simulink library "snn_champions_lib"  (R2026a)
settings: Solver=VariableStepAuto
(part 4 of 24)

== matlab function snn_champions_lib/Michelangelo/SNN ==
  data: x_phys input; params output
function params = SNN(x_phys)
%#codegen
% Blocco champion SELF-CONTAINED: pesi bakati + forward ALIF + decode, zero dipendenze .m.
  W_IN  = [0.5 -0.5 -0.25 2;-1 0.5 -1 2;0.25 -2 1 0.5;0.5 0.25 0.125 -0.25;0.5 -0.5 -0.125 1;-1 1 -1 1;-1 -0.5 0.5 0.5;0.5 0.5 1 -1;-0.25 -0.125 -1 2;-0.5 2 0.25 -0.0625;-0.5 0.0625 0.25 1;0.25 -1 1 1;1 0.5 -0.25 0.125;-2 2 0.5 -0.25;-0.5 1 0.25 -0.5;-0.5 -0.25 1 -1;1 -0.125 0.5 -0.25;0.125 -0.25 2 -0.0625;2 0.0625 -0.25 1;-2 0.5 -0.125 2;0.5 -0.5 1 -0.5;1 0 2 -0.25;-0.25 1 0.25 0.25;1 2 -0.5 -0.125;2 1 -0.5 -0.125;-1 2 0.25 -0.125;0.5 0.5 -0.25 1;-0.5 -0.5 2 -0.0625;1 -0.5 -0.125 0.5;1 -0.0625 0.125 0.5;-0.25 1 0.25 -0.5;-1 1 0.25 0.125];
  U     = [0.125 0 0.0625 0.0625 -0.0625 -0.125 0 0 0.0625 0.0625 0 0.125 0.125 0.0625 -0.125 -0.0625;0 -0.0625 0.0625 -0.0625 0 -0.125 0.0625 -0.0625 0.0625 -0.0625 0 -0.125 0.0625 -0.0625 -0.0625 0;0.0625 0.125 -0.0625 0.0625 0.0625 0.0625 0.0625 0 -0.0625 0 0 0 0.0625 0 0 0.0625;0 0.0625 -0.0625 0.0625 0 -0.0625 0 0 0.0625 -0.0625 -0.0625 0 0.125 0.0625 -0.0625 0.0625;-0.0625 0.0625 0.0625 0 -0.0625 0 -0.0625 0.0625 -0.0625 -0.0625 0 -0.125 0 0.0625 0 0;-0.0625 0.125 -0.125 0 0.0625 -0.125 0.0625 0 0.0625 -0.125 0 -0.0625 0.125 -0.125 -0.125 0;0 -0.0625 -0.125 0 0.125 0.0625 0.0625 0.125 0 -0.0625 -0.0625 0.125 0 -0.125 0 0;-0.0625 0.125 -0.0625 0.125 0.0625 -0.25 0 -0.0625 -0.125 -0.125 -0.125 0.0625 0.0625 -0.125 -0.125 0;0 0.0625 0.0625 -0.125 -0.125 0 0 0 0 -0.0625 -0.0625 0 0 -0.0625 -0.0625 0;0 -0.0625 -0.0625 -0.125 -0.0625 -0.0625 0.0625 0 -0.0625 -0.0625 0 -0.0625 0 0.0625 0 -0.125;0 0.0625 0 -0.125 0 0 -0.0625 0.0625 0 -0.0625 0.0625 0.0625 -0.0625 -0.0625 -0.0625 0.0625;0 0.125 -0.125 0 0.125 0 -0.0625 0.125 -0.125 -0.0625 0 0.0625 0 0 0.0625 0;0 0 0 0 -0.0625 0.0625 0 0.125 0.125 -0.125 0 0.0625 0.0625 0.0625 -0.125 0;-0.0625 0 -0.0625 0 -0.0625 -0.0625 0 -0.25 0 -0.125 0 0.25 0.125 -0.0625 -0.125 0.25;0.0625 0 -0.0625 0 0 -0.0625 0 0 -0.0625 -0.0625 0 0.125 0.125 -0.0625 -0.0625 -0.25;0 0 0.0625 -0.0625 0.0625 -0.125 0.0625 0 0 0.0625 -0.0625 0 0 -0.125 0.0625 0;-0.0625 0.0625 -0.125 0.125 0 -0.125 0.125 0 -0.0625 -0.0625 -0.125 0.0625 0.25 -0.0625 -0.125 -0.125;0 0.0625 -0.0625 0 0 0 0 -0.0625 0 0 -0.0625 0 0 -0.0625 0 0;0 0 0 -0.0625 0 -0.0625 0 0.125 0 -0.0625 0.0625 0 0.125 0.0625 0 -0.125;0.0625 0 0.0625 -0.0625 -0.0625 0 0.25 0.125 0.125 -0.125 -0.125 -0.0625 -0.0625 -0.0625 -0.0625 0.0625;0.125 -0.0625 -0.0625 -0.0625 0.125 0.0625 0 0.0625 -0.0625 0 -0.0625 0.0625 0 0.25 0.0625 0.125;0.0625 0.125 0.125 0.0625 -0.0625 0 0 0 0.125 0 0.0625 0.0625 0 0 0 0.0625;0.25 0 -0.0625 0 -0.125 0.0625 0.125 0 0.0625 -0.125 0 0.0625 -0.25 0.125 0 0.125;0.0625 -0.0625 -0.125 0 -0.125 -0.125 0 0.125 0 0 0 0.25 0 -0.0625 -0.125 0.25;0 -0.125 -0.125 0.125 -0.125 0 0 0.0625 0.125 -0.125 -0.0625 -0.0625 0.125 -0.0625 0.0625 -0.125;-0.0625 0 0.0625 -0.0625 0 -0.25 0 0.0625 0 -0.0625 0 -0.0625 0.0625 0.0625 0.0625 -0.25;0.0625 0.125 -0.0625 0.0625 -0.0625 0.125 0.0625 0.0625 0.0625 -0.0625 0.125 0.0625 -0.0625 -0.0625 0 0;0.0625 0.0625 0 0.125 -0.125 0 -0.0625 -0.125 0 0 -0.125 0.0625 0.0625 0.0625 -0.125 0.125;-0.0625 0 0 0 0.0625 0.0625 0.0625 0.125 -0.0625 -0.125 -0.125 0.0625 0 0 0 0;-0.0625 0.0625 0.125 0.0625 -0.0625 -0.0625 0 0.0625 -0.0625 0 -0.0625 0 0 -0.125 -0.0625 0;0.125 0 0.0625 0 -0.0625 0 0.0625 -0.0625 0.0625 -0.0625 -0.125 0.25 0.125 0.0625 0 0.125;0 0.125 -0.0625 -0.125 0 -0.25 0.0625 0 0 -0.125 0.0625 0 0 0 0.125 0.125];
  V     = [-0.0625 0 0 -0.0625 -0.0625 0 0.5 0.0625 -0.0625 0 0 0.125 -0.0625 -0.125 -0.0625 -0.125 0.25 -0.25 -0.125 0.125 -0.0625 -0.125 -0.0625 -0.0625 0 0 -0.125 0 0.0625 -0.25 -0.125 -0.0625;0.0625 -0.125 0.0625 -0.125 -0.0625 0.125 -0.125 -0.125 -0.25 0.125 -0.125 -0.125 0 -0.0625 0.0625 0.0625 0 -0.125 -0.0625 -0.125 0 0 -0.0625 0.0625 -0.0625 0.125 0 -0.0625 0 0.25 -0.0625 0;-0.125 0.125 0.125 -0.0625 -0.0625 0 0 0.125 0.125 -0.0625 -0.125 0 -0.25 0 0.0625 0.125 -0.125 -0.0625 0 0.25 0.0625 0 -0.0625 0 -0.0625 0 -0.0625 0.0625 -0.125 0 -0.125 0;-0.0625 0 0 0 0.0625 -0.5 -0.125 0 0.125 0 0.0625 -0.0625 0.0625 -0.25 -0.0625 -0.0625 -0.0625 0.125 0.25 -0.125 0 0 -0.0625 0.25 0.25 -0.0625 0 -0.125 -0.125 0.125 0 -0.125;0.125 0 0.125 -0.125 0.125 0.25 0.25 -0.125 0.0625 0.0625 0 0.0625 0.0625 0 0 0 0.125 0 0 -0.25 -0.125 0.0625 0.0625 0.125 0.0625 -0.0625 0.0625 -0.0625 -0.0625 0.125 0 -0.125;0.25 0.125 0 0.0625 0.0625 0.25 -0.0625 -0.0625 0.125 -0.125 0 0.125 0.0625 -0.25 -0.125 0 0.125 0.125 0.125 0.0625 0 0.25 -0.0625 -0.0625 0.0625 -0.125 0 0.0625 0.125 0.25 -0.125 0;-0.0625 0 -0.0625 0.125 -0.0625 0.125 0.0625 -0.0625 0.125 0 -0.0625 0 0.0625 -0.0625 0 0 0 -0.0625 0 0.25 -0.125 -0.0625 0 -0.0625 -0.0625 -0.125 0 -0.125 0.0625 -0.0625 0 -0.125;0 0.25 -0.0625 -0.25 -0.0625 -0.25 0.0625 -0.25 0.125 -0.125 0.125 -0.125 -0.25 0 -0.0625 -0.0625 -0.25 0.5 0 -0.25 -0.125 -0.0625 0.0625 -0.0625 -0.0625 -0.0625 0 0.125 -0.25 -0.125 0.125 0.0625;0.125 0.125 0.125 -0.0625 0.0625 0.25 -0.0625 -0.0625 0.125 -0.25 0.0625 0.0625 0.0625 0 -0.0625 -0.25 0 -0.125 -0.0625 0.125 -0.0625 0 -0.125 -0.125 -0.125 -0.0625 -0.125 0 0.125 0.0625 -0.125 -0.25;-0.125 0.0625 -0.125 0 -0.125 -0.25 0.0625 0.125 0.125 0.0625 0.0625 -0.0625 -0.0625 -0.125 -0.125 -0.0625 0.0625 0.125 0.125 0.0625 0.125 0.125 0.0625 0.125 0.25 0 -0.0625 0.25 0.0625 -0.0625 0.25 -0.0625;-0.0625 0.0625 -0.125 0.25 0 0 -0.0625 0.0625 -0.125 -0.0625 0 0.0625 -0.125 0.125 0.125 -0.0625 0.0625 0.125 -0.125 0 -0.0625 0.125 -0.0625 0 -0.125 0.0625 0 0.125 -0.125 -0.125 0.0625 -0.0625;-0.125 -0.125 -0.0625 -0.0625 0 -0.125 -0.0625 -0.125 -0.125 0 -0.0625 -0.0625 0.0625 -0.0625 0 -0.25 -0.0625 -0.125 -0.125 -0.125 0 0 0 -0.0625 -0.0625 0.125 -0.0625 -0.0625 0 -0.0625 -0.0625 -0.0625;0.125 0.125 0 0.0625 0.125 -0.125 0 0 0 -0.0625 0.125 -0.0625 -0.25 0 -0.0625 -0.125 0 0.0625 0.125 0 -0.0625 -0.0625 -0.0625 0.0625 0.125 -0.0625 -0.0625 0.0625 0 -0.0625 -0.0625 0.0625;0.25 -0.125 0 0.0625 0.0625 0 0 -0.0625 -0.25 0.0625 0 0 0.125 0.0625 0.125 -0.125 0.125 0 0.0625 -0.125 0.25 -0.0625 0.125 0.0625 0 0 0.125 0.0625 -0.0625 0.0625 -0.0625 0;0 -0.25 0.125 0.0625 -0.0625 -0.125 0 0.0625 -0.25 0.125 -0.0625 0.0625 0 0.25 0.0625 -0.125 0.0625 -0.0625 -0.0625 0.0625 0 0.0625 0.125 0 0.0625 0.25 0.125 0 0.0625 0.0625 -0.0625 0.0625;-0.25 0.0625 -0.0625 -0.0625 -0.125 -0.125 -0.125 -0.125 0.125 -0.0625 -0.125 -0.125 -0.125 0 0 0.125 -0.125 -0.0625 0 -0.125 -0.125 0.125 -0.125 0.0625 0.125 -0.125 0 -0.125 -0.125 -0.125 -0.125 -0.125];
  DEL   = [3 5 1 2;2 4 4 4;2 4 0 4;5 0 5 5;1 2 2 2;4 1 4 2;0 4 0 1;0 1 0 1;2 2 1 3;1 2 5 2;0 5 1 2;0 5 3 1;2 0 0 4;2 2 3 4;4 4 5 0;4 5 0 2;0 4 4 3;5 5 4 2;4 5 4 2;3 0 3 1;3 2 0 4;0 4 2 0;5 4 5 2;4 4 3 3;5 3 4 5;2 2 3 1;3 3 5 3;1 3 0 3;1 0 3 2;2 3 4 4;2 4 5 0;1 2 4 0];
  BTH   = [0.55734604597091675;2.1507437229156494;1.1244419813156128;0.14289717376232147;1.9518455266952515;1.3053315877914429;0.37153390049934387;1.0129449367523193;1.2149283885955811;4.9215493202209473;1.1093190908432007;0.84861880540847778;1.7002091407775879;1.749392032623291;1.5353392362594604;0.238857701420784;0.70270282030105591;0.74105638265609741;2.4139764308929443;1.5129112005233765;0.27686840295791626;0.95079588890075684;0.92958110570907593;1.8094992637634277;2.1261751651763916;3.5414290428161621;1.9645473957061768;0.58331090211868286;1.0450270175933838;0.80956119298934937;0.61937046051025391;1.4108703136444092];
  TJ    = [0.49887645244598389;0.49887645244598389;0.49887645244598389;0.49887645244598389;0.49887645244598389;0.49887645244598389;0.49887645244598389;0.49887645244598389;0.49887645244598389;0.49887645244598389;0.49887645244598389;0.49887645244598389;0.49887645244598389;0.49887645244598389;0.49887645244598389;0.49887645244598389;0.49887645244598389;0.49887645244598389;0.49887645244598389;0.49887645244598389;0.49887645244598389;0.49887645244598389;0.49887645244598389;0.49887645244598389;0.49887645244598389;0.49887645244598389;0.49887645244598389;0.49887645244598389;0.49887645244598389;0.49887645244598389;0.49887645244598389;0.49887645244598389];
  LD    = [8;8;8;8;8;8;8;8;8;8;8;8;8;8;8;8;8;8;8;8;8;8;8;8;8;8;8;8;8;8;8;8];
  W_OUT = [0.125 1 -0.25 -0.25 0.0625 2 0.25 -0.5 0.5 1 0.5 0.125 0.5 0.5 0.25 -0.0625 -0.5 -1 0.25 1 -0.5 0.0625 0.5 0.5 0 1 0.5 -0.5 0.25 0.0625 0.25 0.5;0.125 -0.0625 0.0625 0.0625 0.125 -0.25 -0.25 0 0 -0.125 -0.125 0.0625 0.125 -0.5 -0.125 -0.0625 0.125 -0.25 0.25 -0.5 -0.0625 -0.0625 -0.125 0.25 0.25 -0.25 0.0625 -0.25 0.25 0.125 -0.0625 -0.125;-0.125 0.125 -0.5 -0.0625 0 0.0625 -0.5 -0.5 1 0.25 -0.125 -0.5 0.25 0.5 0 -0.5 -0.25 -0.25 0.5 -0.25 -0.25 -0.5 -0.125 0.25 1 0.5 0 -0.125 0.25 -0.25 0.25 0.25;0.125 0.25 0.125 -0.0625 0.125 0.25 0.125 -0.125 0.125 -1 0.0625 0.0625 -0.25 -1 -0.5 -0.25 -0.0625 0.25 0.25 0.0625 0.0625 0 -0.25 -0.25 -0.125 -2 -0.25 0.125 -0.125 0 -0.125 -0.5;0.5 -0.5 0 0.0625 0.25 -0.5 -0.25 -0.0625 -0.25 -0.0625 -0.0625 0 0.125 -0.125 0 -0.125 0.125 -0.25 0.25 -0.5 -0.0625 -0.0625 -0.0625 0.125 0.25 -0.0625 0.125 -0.25 0.125 0.125 -0.0625 0];
  P_LO  = [8;0.5;1;0.30000001192092896;0.5];
  P_HI  = [45;2.5;5;2.5;3];
  D_OFF = [-0.40403744578361511;-0.39011931419372559;1.7717548608779907;2.6884191036224365;-0.95577722787857056];
  L_TAU = [10;3;10;3;3];
  NRM   = [150;40;20;40];
  NT = 10; MAXD = 6; H = size(W_IN, 1);
  % --- normalizzazione (fisico -> [0,1]) ---
  xin = x_phys(:);
  dvc = min(max(xin(3), -NRM(3)), NRM(3));
  xn  = [xin(1)/NRM(1); xin(2)/NRM(2); (dvc + NRM(3))/(2*NRM(3)); xin(4)/NRM(4)];
  % --- stato persistente (registri del blocco) ---
  persistent Vm fat sprev Vli xbuf started
  if isempty(started)
    Vm = zeros(H,1); fat = zeros(H,1); sprev = zeros(H,1);
    Vli = zeros(5,1); xbuf = zeros(4, MAXD); started = true;
  end
  % --- NT tick SNN interni ---
  for k = 1:NT
    xbuf(:, 2:end) = xbuf(:, 1:end-1); xbuf(:, 1) = xn;
    Iin = zeros(H, 1);
    for dd = 0:MAXD-1
      mask = double(DEL == dd);
      Iin = Iin + (W_IN .* mask) * xbuf(:, dd+1);
    end
    rec = U * (V * sprev);
    Vm  = Vm - Vm ./ LD + Iin + rec;
    eth = BTH + max(fat, 0);
    s   = double(Vm >= eth);
    fat = fat - fat ./ LD + s .* max(TJ, 0);
    Vm  = Vm - s .* eth;
    sprev = s;
    Vli = Vli - Vli ./ 8 + W_OUT * s;
  end
  % --- decode -> 5 parametri fisici ---
  adj = (Vli - D_OFF) ./ L_TAU;
  params = P_LO + (P_HI - P_LO) .* (1 ./ (1 + exp(-adj)));
end
